simulink model "PFC_dq_2019_temporelle_etendu"  (R2023a)
settings: Solver=VariableStepAuto  StartTime=0.0  StopTime=temp_simu  RelTol=Te/20
undefined symbols (not defined in the file): C, K_udc_etendu, L, r, Rch, Te, Ud, Udc_cons, Uq, w
libraries: cstblocks x2
settings Model: Creator=xshi  LastModifiedBy=dougl
settings SolverCC: AlgebraicLoopSolver=TrustRegion
settings DebuggingCC: UnconnectedInputMsg=warning  UnconnectedOutputMsg=warning  UnconnectedLineMsg=warning
settings ModelReferenceCC: EnableRefExpFcnMdlSchedulingChecks=on
settings SFSimCC: CustomCodeUndefinedFunction=UseInterfaceOnly

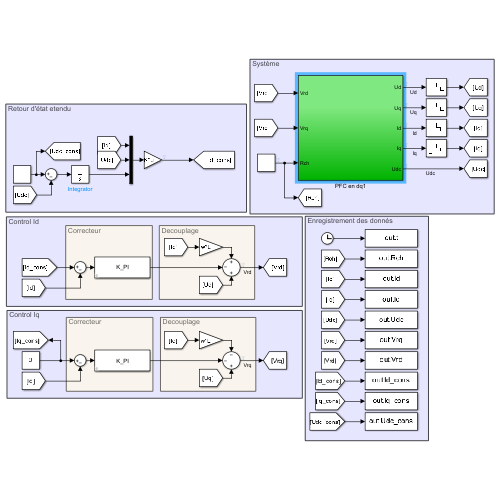
[thumbnail: Simulink's stored preview of the top-level diagram]
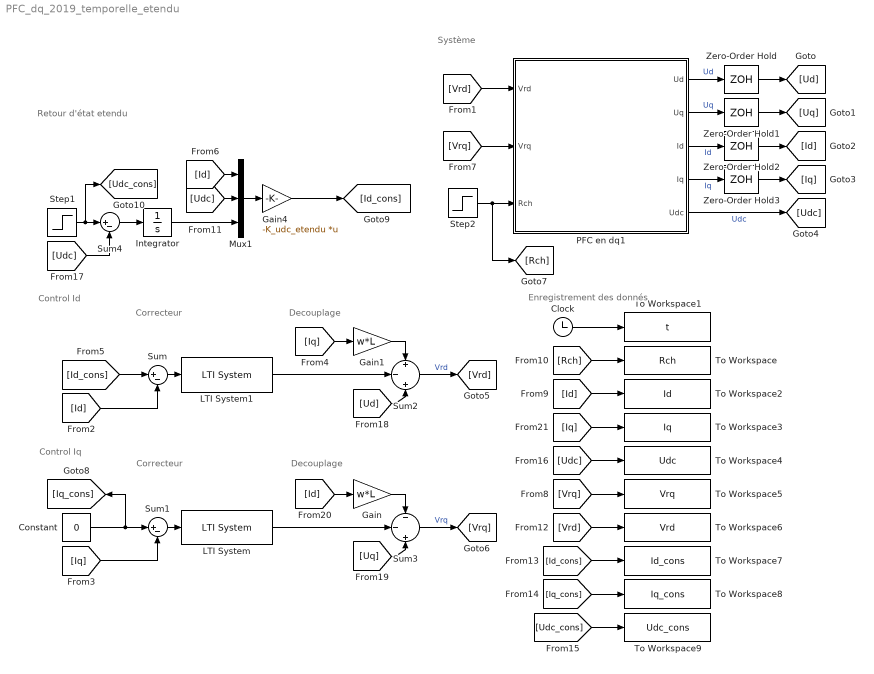
== system PFC_dq_2019_temporelle_etendu ==
  note: Retour d'état etendu
  note: Correcteur
  note: Control Iq
  note: Decouplage
  note: Correcteur
  note: Control Id
  note: Decouplage
  note: Enregistrement des donnés
  note: Système
  Clock : Clock
  Constant : Constant  Value=0  SampleTime=-1
  Gain : Gain  Gain=w*L
  Gain1 : Gain  Gain=w*L
  Gain4 : Gain  Gain=-K_udc_etendu  Multiplication=Matrix(K*u)
  Integrator : Integrator
  LTI System : cstblocks/LTI System  sys=K_PI  IC=[]
  LTI System1 : cstblocks/LTI System  sys=K_PI  IC=[]
  Mux1 : Mux  Inputs=3
  PFC en dq1 : Subsystem
  Step1 : Step  Time=0  After=Udc_cons  SampleTime=0
  Step2 : Step  Time=2.5  Before=Rch  After=Rch/2  SampleTime=0
  Sum : Sum  Inputs=|+-
  Sum1 : Sum  Inputs=|+-
  Sum2 : Sum  Inputs=+|-|+
  Sum3 : Sum  Inputs=-|-|+
  Sum4 : Sum  Inputs=|+-
  To Workspace : ToWorkspace  VariableName=Rch  SampleTime=Te
  To Workspace1 : ToWorkspace  VariableName=t  SampleTime=Te
  To Workspace2 : ToWorkspace  VariableName=Id  SampleTime=Te
  To Workspace3 : ToWorkspace  VariableName=Iq  SampleTime=Te
  To Workspace4 : ToWorkspace  VariableName=Udc  SampleTime=Te
  To Workspace5 : ToWorkspace  VariableName=Vrq  SampleTime=Te
  To Workspace6 : ToWorkspace  VariableName=Vrd  SampleTime=Te
  To Workspace7 : ToWorkspace  VariableName=Id_cons  SampleTime=Te
  To Workspace8 : ToWorkspace  VariableName=Iq_cons  SampleTime=Te
  To Workspace9 : ToWorkspace  VariableName=Udc_cons  SampleTime=Te
  Zero-Order Hold{,1..3} (4 alike) : ZeroOrderHold  SampleTime=Te
  wires:
  Step1/1 -> Sum4/1, [Udc_cons]
  Mux1/1 -> Gain4/1
  [Udc] -> Mux1/2
  [Id] -> Mux1/1
  [Udc] -> Sum4/2
  Sum4/1 -> Integrator/1
  Sum2/1 -> [Vrd]  "Vrd"
  [Id] -> Sum/2
  [Id] -> Gain/1
  [Iq] -> Gain1/1
  LTI System/1 -> Sum3/2
  [Uq] -> Sum3/3
  Sum/1 -> LTI System1/1
  Sum1/1 -> LTI System/1
  Gain/1 -> Sum3/1
  Constant/1 -> Sum1/1, [Iq_cons]
  [Iq] -> Sum1/2
  LTI System1/1 -> Sum2/2
  Gain1/1 -> Sum2/1
  Sum3/1 -> [Vrq]  "Vrq"
  [Id_cons] -> Sum/1
  [Ud] -> Sum2/3
  [Vrq] -> PFC en dq1/2(Vrq)
  Zero-Order Hold3/1 -> [Iq]
  [Vrd] -> PFC en dq1/1(Vrd)
  PFC en dq1/2(Uq) -> Zero-Order Hold1/1  "Uq"
  [Id] -> To Workspace2/1
  [Id_cons] -> To Workspace7/1
  [Udc_cons] -> To Workspace9/1
  [Iq_cons] -> To Workspace8/1
  [Udc] -> To Workspace4/1
  PFC en dq1/1(Ud) -> Zero-Order Hold/1  "Ud"
  [Rch] -> To Workspace/1
  Clock/1 -> To Workspace1/1
  Zero-Order Hold/1 -> [Ud]
  [Vrd] -> To Workspace6/1
  Step2/1 -> [Rch], PFC en dq1/3(Rch)
  PFC en dq1/3(Id) -> Zero-Order Hold2/1  "Id"
  [Iq] -> To Workspace3/1
  [Vrq] -> To Workspace5/1
  PFC en dq1/4(Iq) -> Zero-Order Hold3/1  "Iq"
  Zero-Order Hold2/1 -> [Id]
  Zero-Order Hold1/1 -> [Uq]
  PFC en dq1/5(Udc) -> [Udc]  "Udc"
  Integrator/1 -> Mux1/3
  Gain4/1 -> [Id_cons]

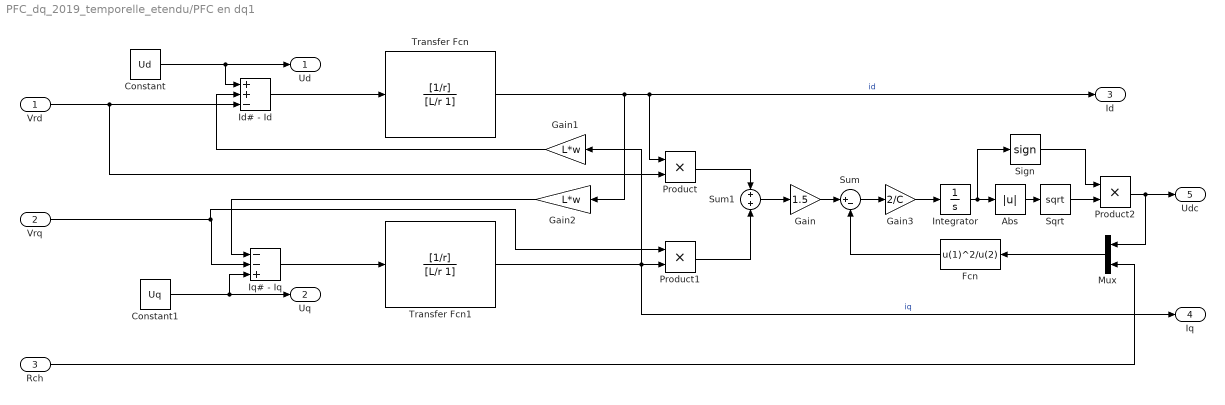
== system PFC_dq_2019_temporelle_etendu/PFC en dq1 ==
  Vrd : Inport
  Vrq : Inport  Port=2
  Rch : Inport  Port=3
  Abs : Abs  SaturateOnIntegerOverflow=off
  Constant : Constant  Value=Ud
  Constant1 : Constant  Value=Uq
  Fcn : Fcn  Expr=u(1)^2/u(2)
  Gain : Gain  Gain=1.5
  Gain1 : Gain  Gain=L*w
  Gain2 : Gain  Gain=L*w
  Gain3 : Gain  Gain=2/C
  Id# - Id : Sum  Inputs=++-  InputSameDT=on  SaturateOnIntegerOverflow=on  OutDataTypeStr=Inherit: Same as first input
  Integrator : Integrator  InitialCondition=0^2
  Iq# - Iq : Sum  Inputs=--+  InputSameDT=on  SaturateOnIntegerOverflow=on  OutDataTypeStr=Inherit: Same as first input
  Mux : Mux  Inputs=2
  Product : Product
  Product1 : Product
  Product2 : Product
  Sign : Signum
  Sqrt : Sqrt
  Sum : Sum  Inputs=|+-
  Sum1 : Sum
  Transfer Fcn : TransferFcn  Numerator=[1/r]  Denominator=[L/r 1]
  Transfer Fcn1 : TransferFcn  Numerator=[1/r]  Denominator=[L/r 1]
  Ud : Outport  VectorParamsAs1DForOutWhenUnconnected=off
  Uq : Outport  Port=2  VectorParamsAs1DForOutWhenUnconnected=off
  Id : Outport  Port=3  VectorParamsAs1DForOutWhenUnconnected=off
  Iq : Outport  Port=4  VectorParamsAs1DForOutWhenUnconnected=off
  Udc : Outport  Port=5  VectorParamsAs1DForOutWhenUnconnected=off
  wires:
  Product2/1 -> Udc/1, Mux/1
  Product1/1 -> Sum1/2
  Product/1 -> Sum1/1
  Sum1/1 -> Gain/1
  Constant1/1 -> Iq# - Iq/3, Uq/1
  Iq# - Iq/1 -> Transfer Fcn1/1
  Constant/1 -> Id# - Id/1, Ud/1
  Vrd/1 -> Id# - Id/3, Product/2
  Transfer Fcn/1 -> Gain2/1, Id/1, Product/1  "id"
  Id# - Id/1 -> Transfer Fcn/1
  Gain2/1 -> Iq# - Iq/1
  Gain1/1 -> Id# - Id/2
  Transfer Fcn1/1 -> Iq/1, Product1/2, Gain1/1  "iq"
  Rch/1 -> Mux/2
  Vrq/1 -> Iq# - Iq/2, Product1/1
  Gain/1 -> Sum/1
  Fcn/1 -> Sum/2
  Integrator/1 -> Sign/1, Abs/1
  Sum/1 -> Gain3/1
  Mux/1 -> Fcn/1
  Gain3/1 -> Integrator/1
  Abs/1 -> Sqrt/1
  Sqrt/1 -> Product2/2
  Sign/1 -> Product2/1
